simulink model "Angel_Error"  (R2021a)
settings: Solver=FixedStepAuto  StartTime=0.0  StopTime=10  FixedStep=0.001  RelTol=1e-3
settings Model: Creator=b00105789  LastModifiedBy=b00105789

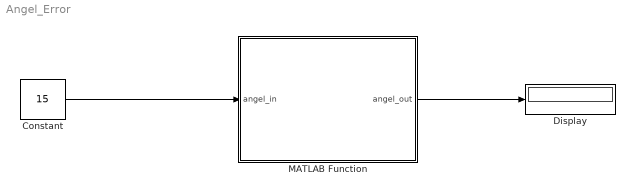
== system Angel_Error ==
  Constant : Constant  Value=15  SampleTime=0.001
  Display : Display
  MATLAB Function : MATLAB Function  TreatAsAtomicUnit=on
  wires:
  Constant/1 -> MATLAB Function/1(angel_in)
  MATLAB Function/1(angel_out) -> Display/1

== matlab function Angel_Error/MATLAB Function ==
  data: angel_in input; angel_out output
function angel_out = angel_error(angel_in)

    N= 10000;
    tol = 1e-9;
    count_real = angel_in/360.000 * N;
   
    if abs(count_real - round(count_real)) < tol
        angel_out = angel_in;
    else
        angel_out = angel_in + 0.006*(angel_in/30);
    end
end
